simulink model "Controllo_cascata_Template_2019"  (R2019b)
settings: Solver=ode1  StartTime=0.0  StopTime=inf  FixedStep=0.002  RelTol=1e-3  EnableMultiTasking=on
PostLoadFcn:
  | qc_set_target_type(getConfigSet(bdroot, 'QUARC Default Target Configuration'));
values from neighbouring files (symbols this model uses):
  den = den{1}    [Km_con_filtri.m]    (also in fft_signal_analysis.m)
  Gden = Gden{1}    [controllore_mag_lin.m]
  Gnum = Gnum{1}    [controllore_mag_lin.m]
  kd = 0    [controller_el.m]    (also in controller_el_windup.m; controllore_el2.m; controllore_mag_lin.m; validation_controller_freq.m)
  ki = 2117.9265    [controller_el.m]    (also in controller_el_windup.m; controllore_el2.m = 104; controllore_mag_lin.m; validation_controller_freq.m = 2118)
  kp = 46.0161    [controller_el.m]    (also in controller_el_windup.m; controllore_el2.m = 0.15; controllore_mag_lin.m; validation_controller_freq.m = 46)
  Lc = 0.3935    [Model_Parameter.m]    (also in Model_Parameter_version2.m = 0.3708; Stima_dei_parametri_Rc_Lc.m = mean(Lc_vect))
  num = num{1}    [Km_con_filtri.m]    (also in fft_signal_analysis.m)
  Rtot = 9.089    [Model_Parameter.m]    (also in Model_Parameter_version2.m = 9.7585)
undefined symbols (not defined in the file or in its folder): den_ext, Gdclose, Gnclose, HIL, num_ext, u0, x10, x1_eq
libraries: simulink x4, quarc_library x4
settings Model: SimulationMode=external  ExtModeTrigDuration=5000  Creator=CFulford  LastModifiedBy=lollo
settings SolverCC: PositivePriorityOrder=on
settings DataIOCC: LimitDataPoints=on  SaveFormat=Array  SignalLoggingSaveFormat=ModelDataLogs  ReturnWorkspaceOutputs=off
settings OptimizationCC: ExpressionDepthLimit=2147483647  InitFltsAndDblsToZero=on  LifeSpan=inf
settings DebuggingCC: SaveWithParameterizedLinksMsg=none  UnderspecifiedInitializationDetection=Classic  MergeDetectMultiDrivingBlocksExec=none  SolverPrmCheckMsg=warning  MultiTaskDSMMsg=warning  MultiTaskCondExecSysMsg=none  FcnCallInpInsideContextMsg=warning  StateNameClashWarn=warning  SFUnexpectedBacktrackingDiag=warning  SFNoUnconditionalDefaultTransitionDiag=warning  SFExecutionAtInitializationDiag=none  ArithmeticOperatorsInVariantConditions=warning
settings HardwareCC: ProdBitPerPointer=32  ProdBitPerSizeT=32  ProdBitPerPtrDiffT=32  ProdLargestAtomicFloat=None  ProdIntDivRoundTo=Undefined  ProdEndianess=Unspecified  ProdWordSize=32  ProdHWDeviceType=32-bit Generic
settings ModelReferenceCC: PropagateSignalLabelsOutOfModel=off
settings SFSimCC: SimUseLocalCustomCode=off  CustomCodeUndefinedFunction=UseInterfaceOnly
settings RTWCC: Description=QUARC Win64 Target  SystemTargetFile=quarc_win64.tlc  TemplateMakefile=quarc_default_tmf  RTWUseLocalCustomCode=off
settings CodeAppCC: StateflowObjectComments=on
settings STFCustomTargetCC: TargetPreCompLibLocation=C:\PROGRA~3\QUARC\lib\2019b\win64\release  ConcurrentExecutionCompliant=on  CombineOutputUpdateFcns=on  CPPClassGenCompliant=on  SystemTargetFile=quarc_win64.tlc
settings GRTTargetCC: TargetPreCompLibLocation=C:\PROGRA~3\QUARC\lib\2019b\win64\release  TargetLangStandard=C89/C90 (ANSI)  ParMdlRefBuildCompliant=off  CompOptLevelCompliant=off  MatFileLogging=off  UseToolchainInfoCompliant=off  ExtMode=on  ExtModeMexFile=quarc_comm
settings ConfigComp: CovMetricSettings=dw  CovSaveCumulativeToWorkspaceVar=on  CovSaveSingleToWorkspaceVar=on  CovExternalEMLEnable=off  CovSFcnEnable=off

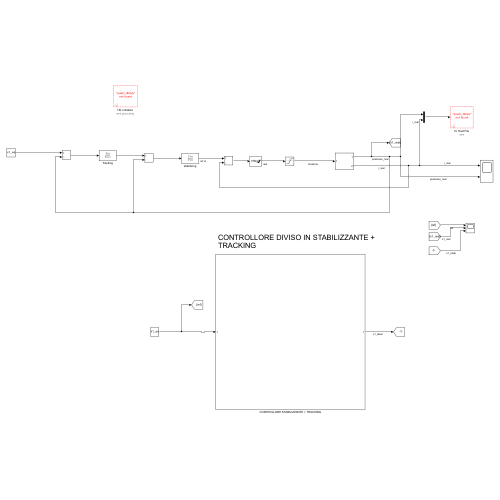
[thumbnail: Simulink's stored preview of the top-level diagram]
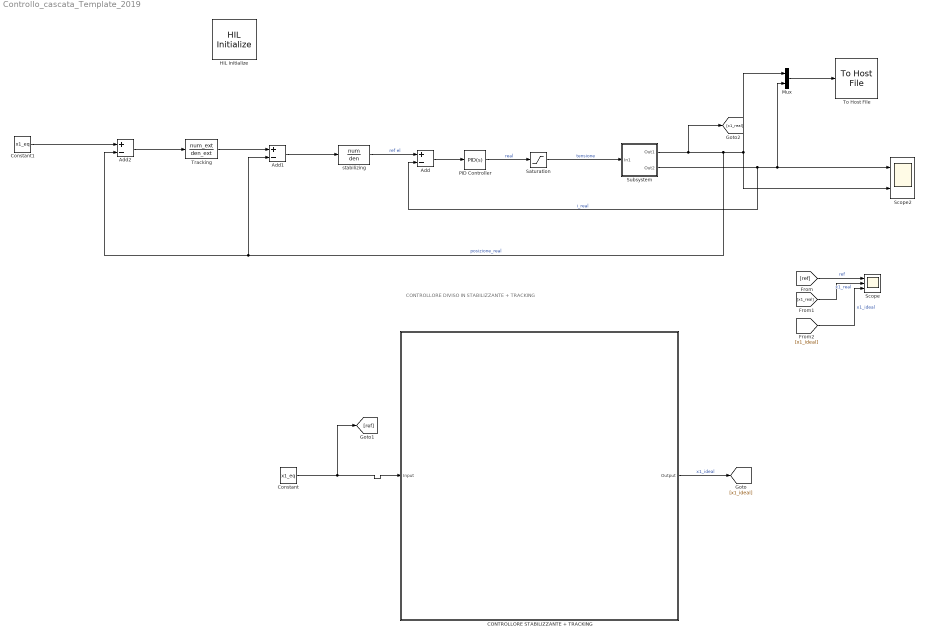
== system Controllo_cascata_Template_2019 ==
  note: CONTROLLORE DIVISO IN STABILIZZANTE + TRACKING
  Add : Sum  Inputs=+-
  Add1 : Sum  Inputs=+-
  Add2 : Sum  Inputs=+-
  CONTROLLORE STABILIZZANTE + TRACKING : Subsystem
  Constant : Constant  Value=x1_eq
  Constant1 : Constant  Value=x1_eq
  HIL Initialize : quarc_library/Data Acquisition/Generic/Configuration/HIL Initialize  Priority=-99  object_name=HIL-1  board_type=q2_usb  board_number=0  board_options=d0=digital;d1=digital;led=auto;update_rate=normal;decimation=1  exclusive=off  active=off  hardware_clocks=[0]  clock_modes=[]  initial_clock_frequencies=[]  set_clock_params_at_start=off  set_clock_params_at_switch_in=off  set_clock_frequencies_at_start=off  set_clock_frequencies_at_switch_in=off  analog_input_channels=[0:1]  analog_input_configurations=[]  analog_input_maximums=10  analog_input_minimums=-10  set_analog_input_params_at_start=on  set_analog_input_params_at_switch_in=off  analog_output_channels=[0:1]  analog_output_maximums=10  analog_output_minimums=-10  initial_analog_outputs=[0]  final_analog_outputs=[0]  watchdog_analog_outputs=0  set_analog_output_params_at_start=on  set_analog_output_params_at_switch_in=off  set_analog_outputs_at_start=on  set_analog_outputs_at_switch_in=off  set_analog_outputs_at_terminate=on  set_analog_outputs_at_switch_out=off  set_analog_outputs_on_watchdog=off  digital_input_channels=[]  digital_output_channels=[]  digital_output_configuration=[]  initial_digital_outputs=[1]  final_digital_outputs=[1]  watchdog_digital_outputs=[1]  set_digital_output_params_at_start=off  set_digital_output_params_at_switch_in=off  set_digital_outputs_at_start=on  set_digital_outputs_at_switch_in=off  set_digital_outputs_at_terminate=on  set_digital_outputs_at_switch_out=off  set_digital_outputs_on_watchdog=off  encoder_channels=[0:1]  quadrature=[4]  encoder_filter_frequency=[]  initial_encoder_counts=[0]  set_encoder_params_at_start=on  set_encoder_params_at_switch_in=off  set_encoder_counts_at_start=on  set_encoder_counts_at_switch_in=off  pwm_channels=[]  pwm_modes=[0]  pwm_frequency=1/0.020  pwm_configuration=[]  pwm_alignment=[]  pwm_polarity=[]  pwm_leading_deadband=[]  pwm_trailing_deadband=[]  initial_pwm_outputs=[0]  final_pwm_outputs=[0]  watchdog_pwm_outputs=[0]  set_pwm_params_at_start=on  set_pwm_params_at_switch_in=off  set_pwm_outputs_at_start=on  set_pwm_outputs_at_switch_in=off  set_pwm_outputs_at_terminate=on  set_pwm_outputs_at_switch_out=off  set_pwm_outputs_on_watchdog=off  other_output_channels=[]  initial_other_outputs=[]  final_other_outputs=[]  watchdog_other_outputs=[]  set_other_outputs_at_start=off  set_other_outputs_at_switch_in=off  set_other_outputs_at_terminate=off  set_other_outputs_at_switch_out=off  set_other_outputs_on_watchdog=off
  Mux : Mux  Inputs=2
  PID Controller : simulink/Continuous/PID Controller  Controller=PID  Form=Parallel  TimeDomain=Continuous-time  SampleTime=-1  IntegratorMethod=Forward Euler  FilterMethod=Forward Euler  ControllerParametersSource=internal  P=kp  I=ki  D=kd  N=100  UseFilter=on  TunerSelectOption=Transfer Function Based (PID Tuner App)  InitialConditionSource=internal  InitialConditionForIntegrator=0  InitialConditionForFilter=0  DifferentiatorICPrevScaledInput=0  ExternalReset=none  TrackingMode=off  Kt=1  LimitOutput=on  UpperSaturationLimit=23  LowerSaturationLimit=-23  LinearizeAsGain=on  AntiWindupMode=clamping  Kb=1  POutMin=[]  POutMax=[]  IOutMin=[]  IOutMax=[]  DOutMin=[]  DOutMax=[]  NOutMin=[]  NOutMax=[]  SumOutMin=[]  SumOutMax=[]  SaturationOutMin=[]  SaturationOutMax=[]  PParamMin=[]  PParamMax=[]  IParamMin=[]  IParamMax=[]  DParamMin=[]  DParamMax=[]  NParamMin=[]  NParamMax=[]  KbParamMin=[]  KbParamMax=[]  KtParamMin=[]  KtParamMax=[]  KbOutMin=[]  KbOutMax=[]  KtOutMin=[]  KtOutMax=[]  IntegratorOutMin=[]  IntegratorOutMax=[]  FilterOutMin=[]  FilterOutMax=[]  SumI1OutMin=[]  SumI1OutMax=[]  SumI2OutMin=[]  SumI2OutMax=[]  SumI3OutMin=[]  SumI3OutMax=[]  SumI4OutMin=[]  SumI4OutMax=[]  SumDOutMin=[]  SumDOutMax=[]  DifferentiatorOutMin=[]  DifferentiatorOutMax=[]  FilterDiffOutCoefMin=[]  FilterDiffOutCoefMax=[]  ReciprocalOutMin=[]  ReciprocalOutMax=[]  SumDenOutMin=[]  SumDenOutMax=[]  SumNumOutMin=[]  SumNumOutMax=[]  DivideOutMin=[]  DivideOutMax=[]  IntegratorContinuousStateAttributes=''  IntegratorStateMustResolveToSignalObject=off  IntegratorRTWStateStorageClass=Auto  FilterContinuousStateAttributes=''  FilterStateMustResolveToSignalObject=off  FilterRTWStateStorageClass=Auto  ParallelPVariant=InternalParameters  IdealPVariant=Disabled  IVariant=InternalParameters  DVariant=InternalParameters  IntegratorVariant=Continuous  SatVariant=Enabled  AWVariant=ContClampingParallel  PCopyVariant=Disabled  TRVariant=Disabled  FdbkBlocksVariant=Forward  IdealPFdbkVariant=Disabled  SatFdbkVariant=Disabled  DerivativeFilterVariant=ContFilter  NVariant=InternalParameters  NCopyVariant=Disabled  FilterICVariant=InternalICsFilter  IntegratorICVariant=InternalICs  ExternalResetVariant=Disabled  TRSumVariant=Passthrough  SumFdbkVariant=Disabled  SumVariant=Sum_PID
  Saturation : Saturate  UpperLimit=23  LowerLimit=-23
  Scope : Scope  NumInputPorts=3
  Scope2 : Scope  NumInputPorts=2
  Subsystem : Subsystem
  To Host File : quarc_library/Sinks/To Host/To Host File  file_name=data_%{date}_%{time}.mat  variable_name=data_%{date}_%{time}  decimation=1  sample_time=-1  file_format=MAT-file v.5  options=No header or footer  append=off  final_file_name=data_25-Mar-2025_18-28-18.mat  bitrate=2000000
  Tracking : TransferFcn  Numerator=num_ext  Denominator=den_ext
  stabilizing : TransferFcn  Numerator=num  Denominator=den
  wires:
  PID Controller/1 -> Saturation/1  "real"
  Add/1 -> PID Controller/1
  Subsystem/1(Out1) -> [x1_real], Add1/2, Add2/2, Mux/1, Scope2/2  "posizione_real"
  Subsystem/2(Out2) -> Add/2, Scope2/1, Mux/2  "i_real"
  Mux/1 -> To Host File/1
  Saturation/1 -> Subsystem/1(In1)  "tensione"
  CONTROLLORE STABILIZZANTE + TRACKING/1(Output) -> [x1_ideal]  "x1_ideal"
  Constant/1 -> [ref], CONTROLLORE STABILIZZANTE + TRACKING/1(Input)
  Tracking/1 -> Add1/1
  Add1/1 -> stabilizing/1
  Add2/1 -> Tracking/1
  Constant1/1 -> Add2/1
  stabilizing/1 -> Add/1  "ref el"
  [ref] -> Scope/1  "ref"
  [x1_real] -> Scope/2  "x1_real"
  [x1_ideal] -> Scope/3  "x1_ideal"

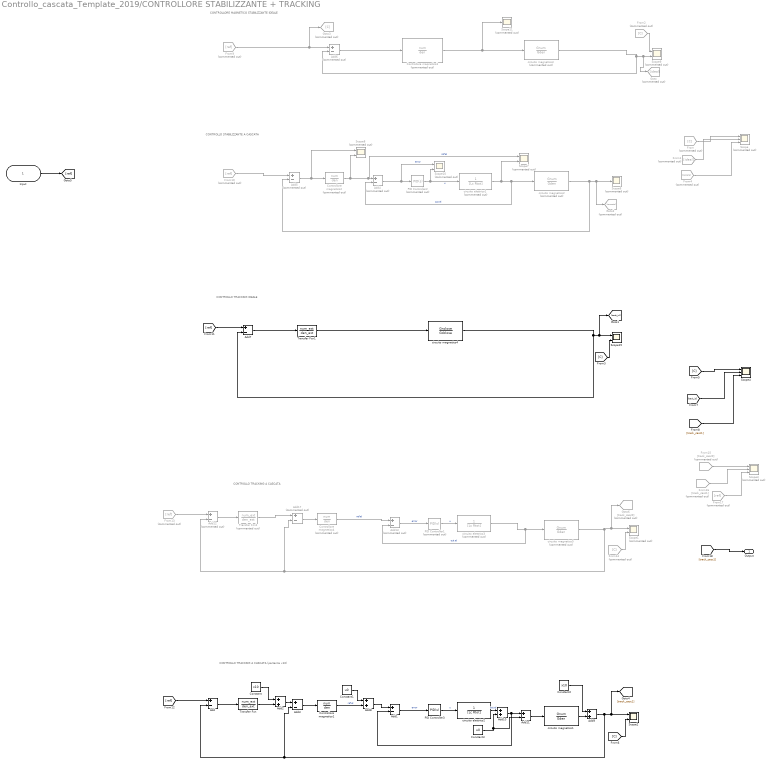
== system Controllo_cascata_Template_2019/CONTROLLORE STABILIZZANTE + TRACKING ==
  note: CONTROLLO STABILIZZANTE A CASCATA
  note: CONTROLLORE MAGNETICO STABILIZZANTE IDEALE
  note: CONTROLLO TRACKING A CASCATA (partenza x10)
  note: CONTROLLO TRACKING IDEALE
  note: CONTROLLO TRACKING A CASCATA
  Input : Inport
  Add{,1,3,7,11} (5 alike) : Sum  Inputs=+-
  Add{2,8..10} (4 alike) : Sum
  Add{4..6,12..13,17} (6 alike) : Sum  Commented=on  Inputs=+-
  Constant : Constant  Value=x10
  Constant1 : Constant  Value=u0
  Constant2 : Constant  Value=x10
  Constant3 : Constant  Value=u0
  Controllore magnetico1 : TransferFcn  Numerator=num  Denominator=den
  Controllore magnetico2 : TransferFcn  Commented=on  Numerator=num  Denominator=den
  Controllore magnetico3 : TransferFcn  Commented=on  Numerator=num  Denominator=den
  Controllore magnetico4 : TransferFcn  Commented=on  Numerator=num  Denominator=den
  From : From  Commented=on  GotoTag=C
  From1 : From  Commented=on  GotoTag=ideal
  From{9..10,13,17} (4 alike) : From  Commented=on  GotoTag=ref
  From14 : From  Commented=on  GotoTag=C
  From15 : From  Commented=on  GotoTag=track_casc0
  From16 : From  Commented=on  GotoTag=track_casc1
  From2 : From  Commented=on  GotoTag=C
  From4 : From  Commented=on  GotoTag=cascata
  Goto : Goto  Commented=on  GotoTag=ideal
  Goto2 : Goto  Commented=on  GotoTag=cascata
  Goto3 : Goto  Commented=on  GotoTag=C
  Goto6 : Goto  Commented=on  GotoTag=track_casc0
  PID Controller1 : simulink/Continuous/PID Controller  Commented=on  Controller=PID  Form=Parallel  TimeDomain=Continuous-time  SampleTime=-1  IntegratorMethod=Forward Euler  FilterMethod=Forward Euler  ControllerParametersSource=internal  P=kp  I=ki  D=0  N=100  UseFilter=on  TunerSelectOption=Transfer Function Based (PID Tuner App)  InitialConditionSource=internal  InitialConditionForIntegrator=0  InitialConditionForFilter=0  DifferentiatorICPrevScaledInput=0  ExternalReset=none  TrackingMode=off  Kt=1  LimitOutput=on  UpperSaturationLimit=23  LowerSaturationLimit=-23  LinearizeAsGain=on  AntiWindupMode=clamping  Kb=1  POutMin=[]  POutMax=[]  IOutMin=[]  IOutMax=[]  DOutMin=[]  DOutMax=[]  NOutMin=[]  NOutMax=[]  SumOutMin=[]  SumOutMax=[]  SaturationOutMin=[]  SaturationOutMax=[]  PParamMin=[]  PParamMax=[]  IParamMin=[]  IParamMax=[]  DParamMin=[]  DParamMax=[]  NParamMin=[]  NParamMax=[]  KbParamMin=[]  KbParamMax=[]  KtParamMin=[]  KtParamMax=[]  KbOutMin=[]  KbOutMax=[]  KtOutMin=[]  KtOutMax=[]  IntegratorOutMin=[]  IntegratorOutMax=[]  FilterOutMin=[]  FilterOutMax=[]  SumI1OutMin=[]  SumI1OutMax=[]  SumI2OutMin=[]  SumI2OutMax=[]  SumI3OutMin=[]  SumI3OutMax=[]  SumI4OutMin=[]  SumI4OutMax=[]  SumDOutMin=[]  SumDOutMax=[]  DifferentiatorOutMin=[]  DifferentiatorOutMax=[]  FilterDiffOutCoefMin=[]  FilterDiffOutCoefMax=[]  ReciprocalOutMin=[]  ReciprocalOutMax=[]  SumDenOutMin=[]  SumDenOutMax=[]  SumNumOutMin=[]  SumNumOutMax=[]  DivideOutMin=[]  DivideOutMax=[]  IntegratorContinuousStateAttributes=''  IntegratorStateMustResolveToSignalObject=off  IntegratorRTWStateStorageClass=Auto  FilterContinuousStateAttributes=''  FilterStateMustResolveToSignalObject=off  FilterRTWStateStorageClass=Auto  ParallelPVariant=InternalParameters  IdealPVariant=Disabled  IVariant=InternalParameters  DVariant=InternalParameters  IntegratorVariant=Continuous  SatVariant=Enabled  AWVariant=ContClampingParallel  PCopyVariant=Disabled  TRVariant=Disabled  FdbkBlocksVariant=Forward  IdealPFdbkVariant=Disabled  SatFdbkVariant=Disabled  DerivativeFilterVariant=ContFilter  NVariant=InternalParameters  NCopyVariant=Disabled  FilterICVariant=InternalICsFilter  IntegratorICVariant=InternalICs  ExternalResetVariant=Disabled  TRSumVariant=Passthrough  SumFdbkVariant=Disabled  SumVariant=Sum_PID
  PID Controller2 : simulink/Continuous/PID Controller  Commented=on  Controller=PID  Form=Parallel  TimeDomain=Continuous-time  SampleTime=-1  IntegratorMethod=Forward Euler  FilterMethod=Forward Euler  ControllerParametersSource=internal  P=kp  I=ki  D=0  N=100  UseFilter=on  TunerSelectOption=Transfer Function Based (PID Tuner App)  InitialConditionSource=internal  InitialConditionForIntegrator=0  InitialConditionForFilter=0  DifferentiatorICPrevScaledInput=0  ExternalReset=none  TrackingMode=off  Kt=1  LimitOutput=on  UpperSaturationLimit=23  LowerSaturationLimit=-23  LinearizeAsGain=on  AntiWindupMode=clamping  Kb=1  POutMin=[]  POutMax=[]  IOutMin=[]  IOutMax=[]  DOutMin=[]  DOutMax=[]  NOutMin=[]  NOutMax=[]  SumOutMin=[]  SumOutMax=[]  SaturationOutMin=[]  SaturationOutMax=[]  PParamMin=[]  PParamMax=[]  IParamMin=[]  IParamMax=[]  DParamMin=[]  DParamMax=[]  NParamMin=[]  NParamMax=[]  KbParamMin=[]  KbParamMax=[]  KtParamMin=[]  KtParamMax=[]  KbOutMin=[]  KbOutMax=[]  KtOutMin=[]  KtOutMax=[]  IntegratorOutMin=[]  IntegratorOutMax=[]  FilterOutMin=[]  FilterOutMax=[]  SumI1OutMin=[]  SumI1OutMax=[]  SumI2OutMin=[]  SumI2OutMax=[]  SumI3OutMin=[]  SumI3OutMax=[]  SumI4OutMin=[]  SumI4OutMax=[]  SumDOutMin=[]  SumDOutMax=[]  DifferentiatorOutMin=[]  DifferentiatorOutMax=[]  FilterDiffOutCoefMin=[]  FilterDiffOutCoefMax=[]  ReciprocalOutMin=[]  ReciprocalOutMax=[]  SumDenOutMin=[]  SumDenOutMax=[]  SumNumOutMin=[]  SumNumOutMax=[]  DivideOutMin=[]  DivideOutMax=[]  IntegratorContinuousStateAttributes=''  IntegratorStateMustResolveToSignalObject=off  IntegratorRTWStateStorageClass=Auto  FilterContinuousStateAttributes=''  FilterStateMustResolveToSignalObject=off  FilterRTWStateStorageClass=Auto  ParallelPVariant=InternalParameters  IdealPVariant=Disabled  IVariant=InternalParameters  DVariant=InternalParameters  IntegratorVariant=Continuous  SatVariant=Enabled  AWVariant=ContClampingParallel  PCopyVariant=Disabled  TRVariant=Disabled  FdbkBlocksVariant=Forward  IdealPFdbkVariant=Disabled  SatFdbkVariant=Disabled  DerivativeFilterVariant=ContFilter  NVariant=InternalParameters  NCopyVariant=Disabled  FilterICVariant=InternalICsFilter  IntegratorICVariant=InternalICs  ExternalResetVariant=Disabled  TRSumVariant=Passthrough  SumFdbkVariant=Disabled  SumVariant=Sum_PID
  PID Controller3 : simulink/Continuous/PID Controller  Controller=PID  Form=Parallel  TimeDomain=Continuous-time  SampleTime=-1  IntegratorMethod=Forward Euler  FilterMethod=Forward Euler  ControllerParametersSource=internal  P=kp  I=ki  D=0  N=100  UseFilter=on  TunerSelectOption=Transfer Function Based (PID Tuner App)  InitialConditionSource=internal  InitialConditionForIntegrator=0  InitialConditionForFilter=0  DifferentiatorICPrevScaledInput=0  ExternalReset=none  TrackingMode=off  Kt=1  LimitOutput=on  UpperSaturationLimit=23  LowerSaturationLimit=-23  LinearizeAsGain=on  AntiWindupMode=clamping  Kb=1  POutMin=[]  POutMax=[]  IOutMin=[]  IOutMax=[]  DOutMin=[]  DOutMax=[]  NOutMin=[]  NOutMax=[]  SumOutMin=[]  SumOutMax=[]  SaturationOutMin=[]  SaturationOutMax=[]  PParamMin=[]  PParamMax=[]  IParamMin=[]  IParamMax=[]  DParamMin=[]  DParamMax=[]  NParamMin=[]  NParamMax=[]  KbParamMin=[]  KbParamMax=[]  KtParamMin=[]  KtParamMax=[]  KbOutMin=[]  KbOutMax=[]  KtOutMin=[]  KtOutMax=[]  IntegratorOutMin=[]  IntegratorOutMax=[]  FilterOutMin=[]  FilterOutMax=[]  SumI1OutMin=[]  SumI1OutMax=[]  SumI2OutMin=[]  SumI2OutMax=[]  SumI3OutMin=[]  SumI3OutMax=[]  SumI4OutMin=[]  SumI4OutMax=[]  SumDOutMin=[]  SumDOutMax=[]  DifferentiatorOutMin=[]  DifferentiatorOutMax=[]  FilterDiffOutCoefMin=[]  FilterDiffOutCoefMax=[]  ReciprocalOutMin=[]  ReciprocalOutMax=[]  SumDenOutMin=[]  SumDenOutMax=[]  SumNumOutMin=[]  SumNumOutMax=[]  DivideOutMin=[]  DivideOutMax=[]  IntegratorContinuousStateAttributes=''  IntegratorStateMustResolveToSignalObject=off  IntegratorRTWStateStorageClass=Auto  FilterContinuousStateAttributes=''  FilterStateMustResolveToSignalObject=off  FilterRTWStateStorageClass=Auto  ParallelPVariant=InternalParameters  IdealPVariant=Disabled  IVariant=InternalParameters  DVariant=InternalParameters  IntegratorVariant=Continuous  SatVariant=Enabled  AWVariant=ContClampingParallel  PCopyVariant=Disabled  TRVariant=Disabled  FdbkBlocksVariant=Forward  IdealPFdbkVariant=Disabled  SatFdbkVariant=Disabled  DerivativeFilterVariant=ContFilter  NVariant=InternalParameters  NCopyVariant=Disabled  FilterICVariant=InternalICsFilter  IntegratorICVariant=InternalICs  ExternalResetVariant=Disabled  TRSumVariant=Passthrough  SumFdbkVariant=Disabled  SumVariant=Sum_PID
  Scope : Scope  Commented=on  NumInputPorts=3
  Scope{1,7..10} (5 alike) : Scope  Commented=on  NumInputPorts=2
  Scope11 : Scope  Commented=on
  Scope15 : Scope  NumInputPorts=2
  Scope2 : Scope  NumInputPorts=2
  Scope3 : Scope  Commented=on  NumInputPorts=3
  Scope4 : Scope  NumInputPorts=3
  Scope6 : Scope  Commented=on
  Transfer Fcn : TransferFcn  Numerator=num_ext  Denominator=den_ext
  Transfer Fcn1 : TransferFcn  Numerator=num_ext  Denominator=den_ext
  Transfer Fcn2 : TransferFcn  Commented=on  Numerator=num_ext  Denominator=den_ext
  circuito elettrico1 : TransferFcn  Commented=on  Denominator=[Lc Rtot]
  circuito elettrico2 : TransferFcn  Denominator=[Lc Rtot]
  circuito elettrico3 : TransferFcn  Commented=on  Denominator=[Lc Rtot]
  circuito magnetico1 : TransferFcn  Numerator=Gnum  Denominator=Gden
  circuito magnetico2 : TransferFcn  Commented=on  Numerator=Gnum  Denominator=Gden
  circuito magnetico3 : TransferFcn  Commented=on  Numerator=Gnum  Denominator=Gden
  circuito magnetico4 : TransferFcn  Numerator=Gnclose  Denominator=Gdclose
  circuito magnetico5 : TransferFcn  Commented=on  Numerator=Gnum  Denominator=Gden
  Output : Outport
  wires:
  circuito magnetico2/1 -> Add5/2, Goto2/1, Scope6/1
  circuito elettrico1/1 -> Scope7/2, Add4/2, circuito magnetico2/1  "out el"
  Add4/1 -> Scope10/1, PID Controller2/1  "error"
  Controllore magnetico2/1 -> Scope8/2, Scope7/1, Add4/1  "ref el"
  PID Controller3/1 -> circuito elettrico2/1  "u"
  [ref] -> Add/1
  Add5/1 -> Scope8/1, Controllore magnetico2/1
  Transfer Fcn1/1 -> circuito magnetico4/1
  Add3/1 -> Controllore magnetico1/1
  Add/1 -> Transfer Fcn/1
  From10/1 -> Add5/1
  circuito magnetico4/1 -> Add7/2, [track_id], Scope15/1
  PID Controller2/1 -> Scope10/2, circuito elettrico1/1  "u"
  Add6/1 -> Controllore magnetico3/1
  From9/1 -> Goto3/1, Add6/1
  circuito magnetico3/1 -> Add6/2, Goto/1, Scope9/2
  Controllore magnetico3/1 -> Scope11/1, circuito magnetico3/1
  Add1/1 -> PID Controller3/1  "error"
  From2/1 -> Scope9/1
  [ref] -> Add7/1
  [C] -> Scope15/2
  Add7/1 -> Transfer Fcn1/1
  [C] -> Scope2/2
  From/1 -> Scope/1
  From1/1 -> Scope/2
  From4/1 -> Scope/3
  [C] -> Scope4/1
  [track_id] -> Scope4/2
  [track_casc1] -> Scope4/3
  Input/1 -> [ref]
  Transfer Fcn/1 -> Add2/2
  Add2/1 -> Add3/1
  Constant/1 -> Add2/1
  Add8/1 -> Add1/1
  Controllore magnetico1/1 -> Add8/2  "ref el"
  Constant1/1 -> Add8/1
  Add9/1 -> [track_casc1], Scope2/1, Add3/2, Add/2
  circuito magnetico1/1 -> Add9/2
  Constant2/1 -> Add9/1
  Add11/1 -> circuito magnetico1/1
  circuito elettrico2/1 -> Add10/1  "out el"
  Add10/1 -> Add1/2, Add11/1
  Constant3/1 -> Add11/2, Add10/2
  From13/1 -> Add12/1
  Controllore magnetico4/1 -> Add13/1  "ref el"
  circuito elettrico3/1 -> Add13/2, circuito magnetico5/1  "out el"
  circuito magnetico5/1 -> Goto6/1, Scope1/1, Add17/2, Add12/2
  Transfer Fcn2/1 -> Add17/1
  Add12/1 -> Transfer Fcn2/1
  From14/1 -> Scope1/2
  Add17/1 -> Controllore magnetico4/1
  PID Controller1/1 -> circuito elettrico3/1  "u"
  Add13/1 -> PID Controller1/1  "error"
  From15/1 -> Scope3/1
  From16/1 -> Scope3/2
  From17/1 -> Scope3/3
  [track_casc1] -> Output/1

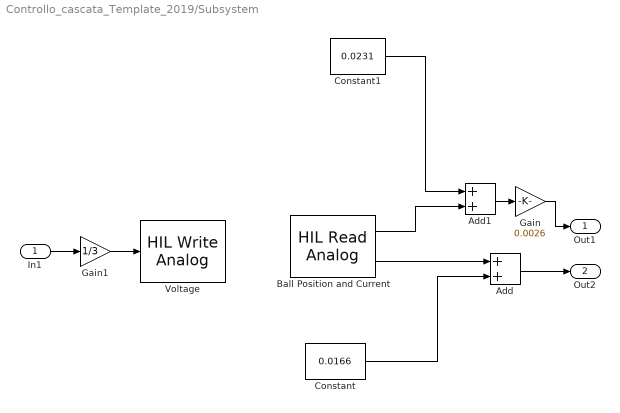
== system Controllo_cascata_Template_2019/Subsystem ==
  In1 : Inport
  Add : Sum
  Add1 : Sum
  Ball Position and Current : quarc_library/Data Acquisition/Generic/Immediate I//O/HIL Read Analog  object_name=HIL-1  channels=[0:1]  sample_time=qc_get_step_size  active=on  vector_output=off
  Constant : Constant  Value=0.0166
  Constant1 : Constant  Value=0.0231
  Gain : Gain  Gain=0.0026
  Gain1 : Gain  Gain=1/3
  Voltage : quarc_library/Data Acquisition/Generic/Immediate I//O/HIL Write Analog  object_name=HIL-1  channels=0  sample_time=-1  active=off  vector_input=off
  Out1 : Outport
  Out2 : Outport  Port=2
  wires:
  In1/1 -> Gain1/1
  Ball Position and Current/1 -> Add1/2
  Ball Position and Current/2 -> Add/1
  Constant/1 -> Add/2
  Constant1/1 -> Add1/1
  Add1/1 -> Gain/1
  Gain/1 -> Out1/1
  Add/1 -> Out2/1
  Gain1/1 -> Voltage/1
